simulink model "model_simulator"  (R2019b)
settings: Solver=FixedStepAuto  StartTime=0.0  StopTime=10.0  FixedStep=0.01  RelTol=1e-3
libraries: dspsigops x1
settings Model: Creator=mchehadeh  LastModifiedBy=Khalil
settings DataIOCC: ReturnWorkspaceOutputs=off
settings DebuggingCC: InheritedTsInSrcMsg=none  ArithmeticOperatorsInVariantConditions=warning
settings SFSimCC: CustomCodeUndefinedFunction=UseInterfaceOnly

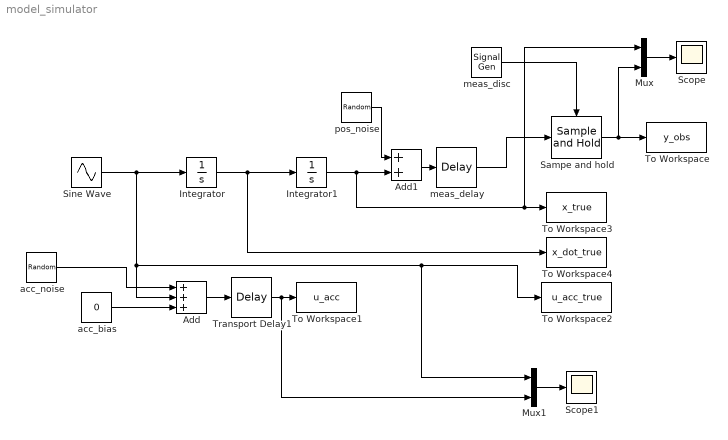
== system model_simulator ==
  Add : Sum  Inputs=+++
  Add1 : Sum
  Integrator : Integrator
  Integrator1 : Integrator
  Mux : Mux  Inputs=2
  Mux1 : Mux  Inputs=2
  Sampe and hold : dspsigops/Sample and Hold  trig=Rising edge  initCond=0  latchinput=off
  Scope : Scope
  Scope1 : Scope
  Sine Wave : Sin  Amplitude=10  Frequency=pi  SampleTime=0
  To Workspace : ToWorkspace  VariableName=y_obs  SaveFormat=Timeseries  SampleTime=-1
  To Workspace1 : ToWorkspace  VariableName=u_acc  SaveFormat=Timeseries  SampleTime=-1
  To Workspace2 : ToWorkspace  VariableName=u_acc_true  SaveFormat=Timeseries  SampleTime=-1
  To Workspace3 : ToWorkspace  VariableName=x_true  SaveFormat=Timeseries  SampleTime=-1
  To Workspace4 : ToWorkspace  VariableName=x_dot_true  SaveFormat=Timeseries  SampleTime=-1
  Transport Delay1 : TransportDelay  DelayTime=0
  acc_bias : Constant  Value=0
  acc_noise : RandomNumber  Variance=0
  meas_delay : TransportDelay  DelayTime=0.04
  meas_disc : SignalGenerator  WaveForm=square  Frequency=50
  pos_noise : RandomNumber  Variance=0
  wires:
  Integrator/1 -> To Workspace4/1, Integrator1/1
  acc_noise/1 -> Add/1
  Integrator1/1 -> Mux/1, To Workspace3/1, Add1/2
  pos_noise/1 -> Add1/1
  Add1/1 -> meas_delay/1
  Add/1 -> Transport Delay1/1
  acc_bias/1 -> Add/3
  meas_delay/1 -> Sampe and hold/1
  Sampe and hold/1 -> Mux/2, To Workspace/1
  meas_disc/1 -> Sampe and hold/Trigger
  Mux/1 -> Scope/1
  Mux1/1 -> Scope1/1
  Sine Wave/1 -> Mux1/1, To Workspace2/1, Add/2, Integrator/1
  Transport Delay1/1 -> Mux1/2, To Workspace1/1
